simulink model "kuvvetler_ve_momentler"  (R2023b)
settings: Solver=VariableStepAuto  StartTime=0.0  StopTime=10000.0  RelTol=1e-3
libraries: sim3dlib x1, uavsim3dlib x1, robotcorelib x1, simulink_extras x1
settings Model: Creator=SafakPC  LastModifiedBy=SafakPC

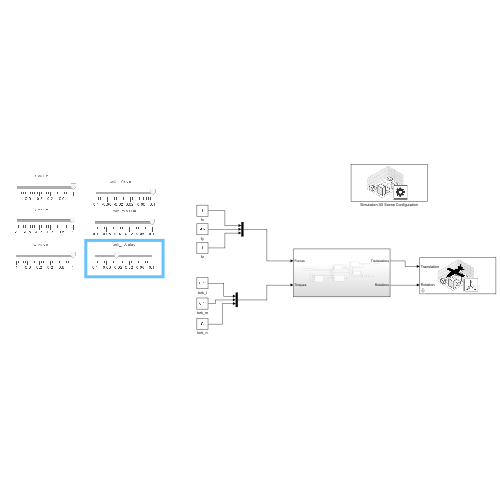
[thumbnail: Simulink's stored preview of the top-level diagram]
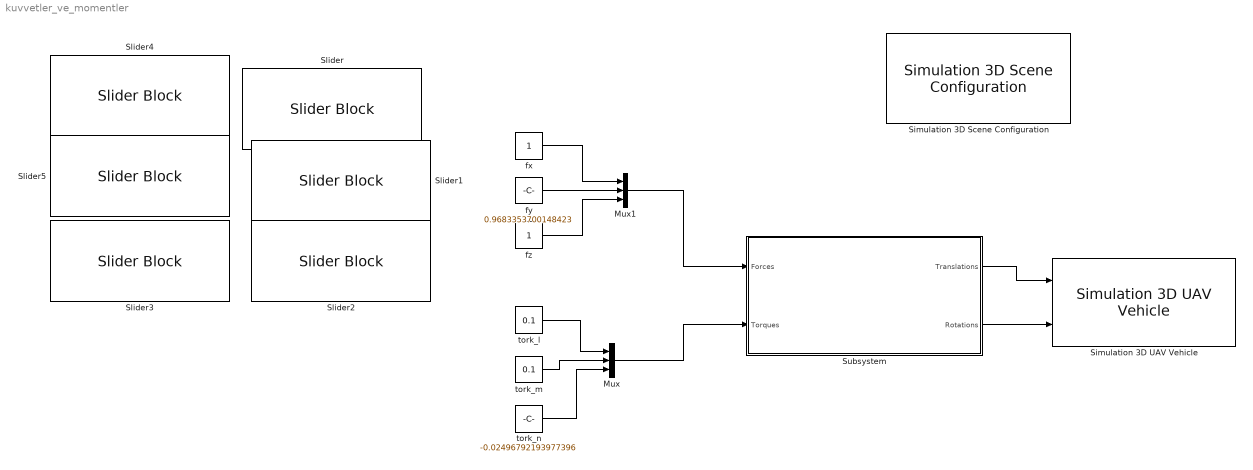
== system kuvvetler_ve_momentler ==
  Mux : Mux  Inputs=3
  Mux1 : Mux  Inputs=3
  Simulation 3D Scene Configuration : sim3dlib/Simulation 3D Scene Configuration  Priority=0  ProjectFormat=Default Scenes  SceneDesc=US city block  ProjectName=C:\Program Files\MATLAB\R2023b\toolbox\shared\sim3d_projects\automotive_project_windows\UE\WindowsNoEditor\VehicleSimulation.exe  ScenePath=/Game/Maps/USCityBlock  EnableOpenDRIVE=off  vehTagList={'Custom';'Scene Origin';'SimulinkVehicle1'}  vehTag=SimulinkVehicle1  FreeCameraInitialTranslation=[0, 0, 0]  FreeCameraDefaultInitialTranslation=[-6, 0, 2]  FreeCameraInitialRotation=[0, 0, 0]  FreeCameraDefaultInitialRotation=[0, -15, 0]  OpVisEn=off  Ts=1/60  EnableWindow=on  EnableRemoteAccess=off  EnableWeather=off  SunAltitude=40.0  SunAzimuth=90  clouds=10  wind=1  fog=0  rain=0  EnableGeospatial=off  OriginHeight=200  OriginLatitude=40.744652  OriginLongitude=-73.988864  MapStyle=Aerial  AdditionalAssetIDs=[]  UseAdvancedSunSky=off  SolarTime=11  TimeZone=-5  Day=21  Month=9  Year=2022  UseDaylightSavingTime=on  DSTStartDay=10  DSTStartMonth=3  DSTEndDay=3  DSTEndMonth=11  DSTSwitchHour=2  sensorTag=MainCamera1  sensorId=1  sensorName=MainCamera1  mountLoc=Origin  offsetFlag=off  tmountOffset=[0, 0, 0]  rmountOffset=[0, 0, 0]  HorizontalResolution=1280  VerticalResolution=720  HorizontalFOV=60  mountPoint=[0 0 0]  mountOrientation=[0 0 0]  aMode=4  ID=1  GeoTrigger=Inactive
      settings: LibrarySourceBlock=uavsim3dlib/Simulation 3D Scene Configuration
  Simulation 3D UAV Vehicle : uavsim3dlib/Simulation 3D UAV Vehicle  Priority=-1  Mesh=Fixed wing  MeshPath=/MathWorksUAVContent/UAVs/HexaRotorUAV/HexaRotor.HexaRotor  Color=Blue  ActorName=SimulinkVehicle1  UseGlobalFrame=off  InitialTranslation=[1000 1000 1000]  InitialRotation=[20 20 20]  InitialTranslationGlobal=[0 0 0]  InitialGeoOrigin=[0 0 0]  InitialRotationGlobal=[0 0 0]  SampleTime=-1  ActorType=SimulinkVehicle  ID=1  aMode=4  ActorTag=SimulinkVehicle1
  Slider : SliderBlock  ScaleMin=-0.1  ScaleMax=0.1
  Slider1 : SliderBlock  ScaleMin=-0.1  ScaleMax=0.1
  Slider2 : SliderBlock  ScaleMin=-0.1  ScaleMax=0.1
  Slider3 : SliderBlock  ScaleMin=-1  ScaleMax=1
  Slider4 : SliderBlock  ScaleMin=-1  ScaleMax=1
  Slider5 : SliderBlock  ScaleMin=-1  ScaleMax=1
  Subsystem : Subsystem
  fx : Constant
  fy : Constant  Value=0.9683353700148423
  fz : Constant
  tork_l : Constant  Value=0.1
  tork_m : Constant  Value=0.1
  tork_n : Constant  Value=-0.02496792193977396
  wires:
  tork_l/1 -> Mux/1
  tork_m/1 -> Mux/2
  tork_n/1 -> Mux/3
  fy/1 -> Mux1/2
  fx/1 -> Mux1/1
  fz/1 -> Mux1/3
  Mux/1 -> Subsystem/2(Torques)
  Mux1/1 -> Subsystem/1(Forces)
  Subsystem/1(Translations) -> Simulation 3D UAV Vehicle/1
  Subsystem/2(Rotations) -> Simulation 3D UAV Vehicle/2

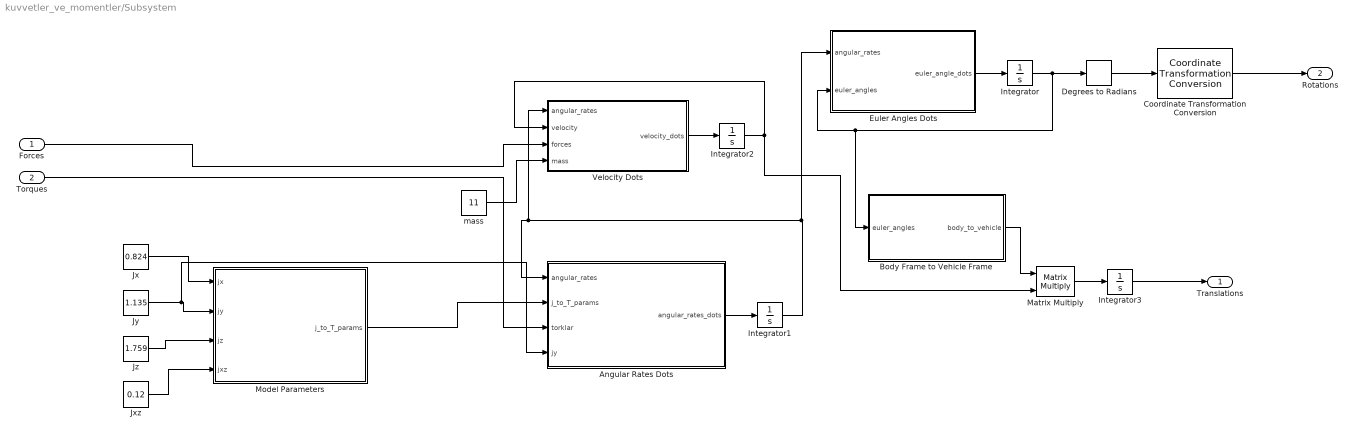
== system kuvvetler_ve_momentler/Subsystem ==
  Forces : Inport
  Torques : Inport  Port=2
  Angular Rates Dots : MATLAB Function  TreatAsAtomicUnit=on
  Body Frame to Vehicle Frame : MATLAB Function  TreatAsAtomicUnit=on
  Coordinate Transformation Conversion : robotcorelib/Coordinate Transformation Conversion  InputRepresentation=Euler Angles  InputEulerSequence=XYZ  ShowTrVecInputPort=on  OutputRepresentation=Quaternion  OutputEulerSequence=ZYX  ShowTrVecOutputPort=on  SimulateUsing=Interpreted execution
      settings: LibrarySourceBlock=uavutilslib/Coordinate Transformation Conversion
  Degrees to Radians : simulink_extras/Transformations/Degrees to Radians
  Euler Angles Dots : MATLAB Function  TreatAsAtomicUnit=on
  Integrator{,1..3} (4 alike) : Integrator
  Jx : Constant  Value=0.824
  Jxz : Constant  Value=0.12
  Jy : Constant  Value=1.135
  Jz : Constant  Value=1.759
  Matrix Multiply : Product  Multiplication=Matrix(*)
  Model Parameters : MATLAB Function  TreatAsAtomicUnit=on
  Velocity Dots : MATLAB Function  TreatAsAtomicUnit=on
  mass : Constant  Value=11
  Translations : Outport
  Rotations : Outport  Port=2
  wires:
  Degrees to Radians/1 -> Coordinate Transformation Conversion/1
  Coordinate Transformation Conversion/1 -> Rotations/1
  Jy/1 -> Angular Rates Dots/4(jy), Model Parameters/2(jy)
  Jxz/1 -> Model Parameters/4(jxz)
  Integrator3/1 -> Translations/1
  Jz/1 -> Model Parameters/3(jz)
  Jx/1 -> Model Parameters/1(jx)
  Model Parameters/1(j_to_T_params) -> Angular Rates Dots/2(j_to_T_params)
  Torques/1 -> Angular Rates Dots/3(torklar)
  mass/1 -> Velocity Dots/4(mass)
  Forces/1 -> Velocity Dots/3(forces)
  Angular Rates Dots/1(angular_rates_dots) -> Integrator1/1
  Integrator1/1 -> Euler Angles Dots/1(angular_rates), Velocity Dots/1(angular_rates), Angular Rates Dots/1(angular_rates)
  Velocity Dots/1(velocity_dots) -> Integrator2/1
  Integrator2/1 -> Matrix Multiply/2, Velocity Dots/2(velocity)
  Euler Angles Dots/1(euler_angle_dots) -> Integrator/1
  Integrator/1 -> Body Frame to Vehicle Frame/1(euler_angles), Euler Angles Dots/2(euler_angles), Degrees to Radians/1
  Matrix Multiply/1 -> Integrator3/1
  Body Frame to Vehicle Frame/1(body_to_vehicle) -> Matrix Multiply/1

== matlab function kuvvetler_ve_momentler/Subsystem/Model Parameters ==
  data: jx input; j_to_T_params output; jy input; jz input; jxz input
function j_to_T_params = fcn(jx,jy,jz,jxz)

T = ((jx*jz)-(jxz*jxz));
T1 = ((jxz)*(jx-jy+jz))/T;
T2 = ((jz*(jz-jy))+(jxz*jxz))/T;
T3 = jz/T;
T4 = jxz/T;
T5 = (jz-jx)/jy;
T6 =jxz/jy;
T7 = (((jx-jy)*jx)+(jxz*jxz))/T;
T8 =jx/T;

j_to_T_params = [T;T1;T2;T3;T4;T5;T6;T7;T8];

end

== matlab function kuvvetler_ve_momentler/Subsystem/Euler Angles Dots ==
  data: angular_rates input size=3; euler_angle_dots output size=3; euler_angles input size=3
function euler_angle_dots = fcn(angular_rates, euler_angles)
    p = angular_rates(1);
    q = angular_rates(2);
    r = angular_rates(3);
    phi = euler_angles(1);
    theta = euler_angles(2);
    psi = euler_angles(3);
    % Matris elemanlarını tanımlama
    a11 = 1;
    a21 = 0;
    a31 = 0;
    a12 = sin(phi)*tan(theta);
    a13 = cos(phi)*tan(theta);
    a22 = cos(phi);
    a23 = -sin(phi);
    a32 = sin(phi)/cos(theta);
    a33 = cos(phi)/cos(theta);
    
    % 3x3 matris
    matris_3x3 = [a11, a12, a13; 
                  a21, a22, a23; 
                  a31, a32, a33];
    
    % 3x1 matris
    matris_3x1 = [p; q; r];
    
    % Matris çarpımı
    euler_angle_dots = matris_3x3 * matris_3x1;
end

== matlab function kuvvetler_ve_momentler/Subsystem/Angular Rates Dots ==
  data: angular_rates input size=3; angular_rates_dots output size=3; j_to_T_params input; torklar input; jy input
function angular_rates_dots = fcn(angular_rates,j_to_T_params,torklar,jy)
    p = angular_rates(1);
    q = angular_rates(2);
    r = angular_rates(3);
    T = j_to_T_params(1);
    T1 = j_to_T_params(2);
    T2 = j_to_T_params(3);
    T3 = j_to_T_params(4);
    T4 = j_to_T_params(5);
    T5 = j_to_T_params(6);
    T6 = j_to_T_params(7);
    T7 = j_to_T_params(8);
    T8 = j_to_T_params(9);
    tork_l = torklar(1);
    tork_m = torklar(2);
    tork_n = torklar(3);
    % Matris elemanlarını tanımlama

    a11 = ((T1*p*q) - (T2*q*r));
    a21 = ((T5*p*r)- (T6*((p*p)-(r*r))));
    a31 =  ((T7*p*q) - (T1*q*r));

    b11 = ((T3*tork_l) + (T4*tork_n));
    b21 = ((1/jy)*tork_m);
    b31 = ((T4*tork_l) + (T8*tork_n));

    m1 = [a11; a21; a31];
    m2 = [b11; b21; b31];

    angular_rates_dots = m1 + m2;

end

== matlab function kuvvetler_ve_momentler/Subsystem/Velocity Dots ==
  data: angular_rates input size=3; velocity_dots output size=3; velocity input; forces input; mass input
function velocity_dots = fcn(angular_rates,velocity,forces,mass)
    p = angular_rates(1);
    q = angular_rates(2);
    r = angular_rates(3);
    u = velocity(1);
    v = velocity(2);
    w = velocity(3);
    fx = forces(1);
    fy = forces(2);
    fz = forces(3);

    a11 = ((r*v) - (q*w));
    a21 = ((p*w) - (r*u));
    a31 = ((q*u) - (p*v));

    m1 = [a11;a21;a31];
    m2 = (1/mass)*[fx;fy;fz];
    m3 = m1+m2;
    
    velocity_dots = m3;

end

== matlab function kuvvetler_ve_momentler/Subsystem/Body Frame to Vehicle Frame ==
  data: euler_angles input size=3; body_to_vehicle output
function body_to_vehicle = fcn(euler_angles)
    phi = euler_angles(1);
    theta = euler_angles(2);
    psi = euler_angles(3);
    % Dönüşüm matrisini oluştur
    body_to_vehicle = [cos(theta)*cos(psi), sin(phi)*sin(theta)*cos(psi) - cos(phi)*sin(psi), cos(phi)*sin(theta)*cos(psi) + sin(phi)*sin(psi);
                       cos(theta)*sin(psi), sin(phi)*sin(theta)*sin(psi) + cos(phi)*cos(psi), cos(phi)*sin(theta)*sin(psi) - sin(phi)*cos(psi);
                       -sin(theta), sin(phi)*cos(theta), cos(phi)*cos(theta)];

end
